simulink model "F16_Real5_OpenLoopSuccessTest_Dai3_NoHDU"  (R2016b)
settings: Solver=ode4  StartTime=0.0  StopTime=35  FixedStep=0.01  RelTol=1e-5  AbsTol=1e-4  EnableMultiTasking=on
InitFcn:
  | F16_Real5_init
libraries: simulink x2, vrlib x1
settings Model: SimulationMode=accelerator  Creator=WhisPer  LastModifiedBy=dream
settings DataIOCC: LimitDataPoints=on  SaveFormat=Array
settings OptimizationCC: LifeSpan=inf
settings DebuggingCC: UnderspecifiedInitializationDetection=Classic  MergeDetectMultiDrivingBlocksExec=none  SolverPrmCheckMsg=warning  StateNameClashWarn=warning  SFUnexpectedBacktrackingDiag=warning  SFNoUnconditionalDefaultTransitionDiag=warning  SFExecutionAtInitializationDiag=none
settings HardwareCC: ProdBitPerPointer=32  ProdBitPerSizeT=32  ProdBitPerPtrDiffT=32  ProdLargestAtomicFloat=None  ProdIntDivRoundTo=Undefined  ProdEndianess=Unspecified  ProdWordSize=32  ProdHWDeviceType=32-bit Generic
settings ModelReferenceCC: PropagateSignalLabelsOutOfModel=off
settings GRTTargetCC: TargetLangStandard=C89/C90 (ANSI)  GeneratePreprocessorConditionals=Disable all
settings ConfigComp: CovMetricSettings=dw  CovHtmlReporting=on  CovSaveCumulativeToWorkspaceVar=on  CovSaveSingleToWorkspaceVar=on  CovExternalEMLEnable=off

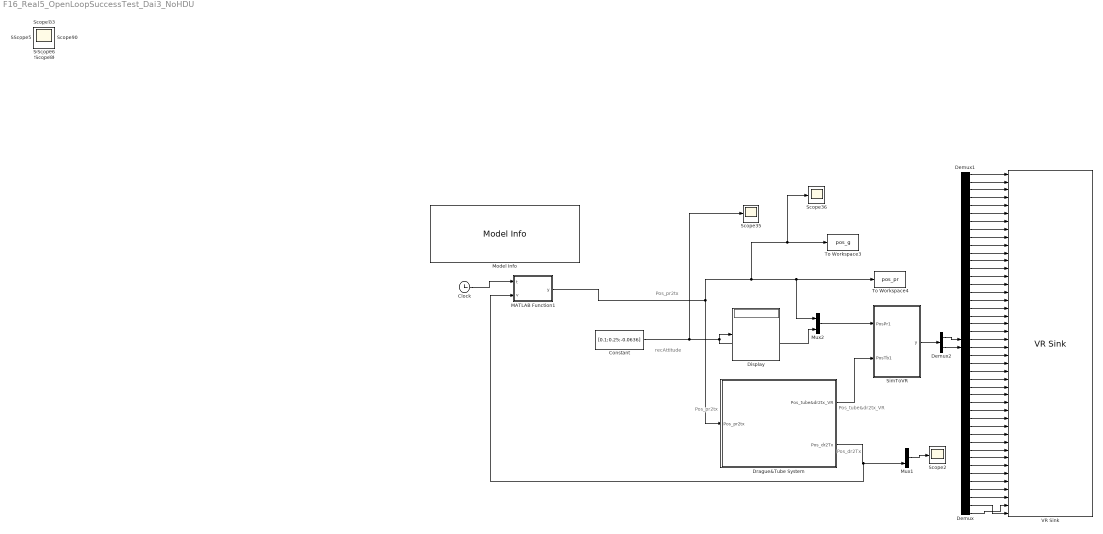
== system F16_Real5_OpenLoopSuccessTest_Dai3_NoHDU ==
  note: recAttitude
  note: Pos_dr2Tx
  note: Pos_tube&dr2tx_VR
  note: Pos_pr2tx
  note: Pos_pr2tx
  Clock : Clock
  Constant : Constant  Value=[0.1;0.25;-0.0636]
  Demux : Demux  Outputs=22
  Demux1 : Demux  Outputs=22
  Demux2 : Demux  Outputs=[88,66]
  Display : Display
  Drague&Tube System : Subsystem
      mask Display: image(imread('Icon\zhuitao.png'))
  MATLAB Function1 : MATLAB Function  TreatAsAtomicUnit=on
  Model Info : simulink/Model-Wide Utilities/Model Info  BlockCM=None  Frame=on  DisplayStringWithTags=|  HorizontalTextAlignment=Center  LeftAlignmentValue=0.5  SourceBlockDiagram=F16_Real5_OpenLoopSuccessTest_Dai3_NoHDU  TagMaxNumber=20
      | Ppr_rc=[6.06 0.54 -0.86]
      | Pns_rc=[8.00 0.00  0.00]
      | Pfl_rc=[3.75 0.00 -0.86]
      | Pdr0_tk=[-13.549 0.00 5]
  Mux1 : Mux  Inputs=2
  Mux2 : Mux  Inputs=2
  Scope{,1..36} (37 alike) : Scope
  SimToVR : MATLAB Function  TreatAsAtomicUnit=on
  To Workspace3 : ToWorkspace  VariableName=pos_g  SampleTime=-1
  To Workspace4 : ToWorkspace  VariableName=pos_pr  SampleTime=-1
  VR Sink : vrlib/VR Sink  InstantiateOnLoad=on  SampleTime=-1  ViewEnable=on  RemoteChange=off  RemoteView=off  FieldsWritten=tube1.rotation.4.1.1.double#tube1.translation.3.1.1.double#tube2.rotation.4.1.1.double#tube2.translation.3.1.1.double#tube3.rotation.4.1.1.double#tube3.translation.3.1.1.double#tube4.rotation.4.1.1.double#tube4.translation.3.1.1.double#tube5.rotation.4.1.1.double#tube5.translation.3.1.1.double#tube6.rotation.4.1.1.double#tube6.translation.3.1.1.double#tube7.rotation.4.1.1.double#tube7.translation.3.1.1.double#tube8.rotation.4.1.1.double#tube8.translation.3.1.1.double#tube9.rotation.4.1.1.double#tube9.translation.3.1.1.double#tube10.rotation.4.1.1.double#tube10.translation.3.1.1.double#tube11.rotation.4.1.1.double#tube11.translation.3.1.1.double#tube12.rotation.4.1.1.double#tube12.translation.3.1.1.double#tube13.rotation.4.1.1.double#tube13.translation.3.1.1.double#tube14.rotation.4.1.1.double#tube14.translation.3.1.1.double#tube15.rotation.4.1.1.double#tube15.translation.3.1.1.double#tube16.rotation.4.1.1.double#tube16.translation.3.1.1.double#tube17.rotation.4.1.1.double#tube17.translation.3.1.1.double#tube18.rotation.4.1.1.double#tube18.translation.3.1.1.double#tube19.rotation.4.1.1.double#tube19.translation.3.1.1.double#tube20.rotation.4.1.1.double#tube20.translation.3.1.1.double#tube21.rotation.4.1.1.double#tube21.translation.3.1.1.double#ASDD.translation.3.1.1.double#Receiver.rotation.4.1.1.double  WorldFileName=AirRefuelingTubeSim.WRL  AutoView=off  VideoDimensions=[]  AllowVariableSize=off
  wires:
  MATLAB Function1/1(y) -> Drague&Tube System/1(Pos_pr2tx), Mux2/1, To Workspace4/1, Scope36/1, To Workspace3/1
  Drague&Tube System/2(Pos_dr2Tx) -> MATLAB Function1/2(v), Mux1/2
  Mux1/1 -> Scope2/1
  Constant/1 -> Scope35/1, Display/1, Mux2/2
  Demux2/2 -> Demux/1
  SimToVR/1(y) -> Demux2/1
  Drague&Tube System/1(Pos_tube&dr2tx_VR) -> SimToVR/2(PosTb1)
  Mux2/1 -> SimToVR/1(PosPr1)
  Demux1/1 -> VR Sink/1
  Demux/1 -> VR Sink/2
  Demux1/2 -> VR Sink/3
  Demux/2 -> VR Sink/4
  Demux1/3 -> VR Sink/5
  Demux/3 -> VR Sink/6
  Demux1/4 -> VR Sink/7
  Demux/4 -> VR Sink/8
  Demux1/5 -> VR Sink/9
  Demux/5 -> VR Sink/10
  Demux1/6 -> VR Sink/11
  Demux/6 -> VR Sink/12
  Demux1/7 -> VR Sink/13
  Demux/7 -> VR Sink/14
  Demux1/8 -> VR Sink/15
  Demux/8 -> VR Sink/16
  Demux1/9 -> VR Sink/17
  Demux/9 -> VR Sink/18
  Demux1/10 -> VR Sink/19
  Demux/10 -> VR Sink/20
  Demux1/11 -> VR Sink/21
  Demux/11 -> VR Sink/22
  Demux1/12 -> VR Sink/23
  Demux/12 -> VR Sink/24
  Demux1/13 -> VR Sink/25
  Demux/13 -> VR Sink/26
  Demux1/14 -> VR Sink/27
  Demux/14 -> VR Sink/28
  Demux1/15 -> VR Sink/29
  Demux/15 -> VR Sink/30
  Demux1/16 -> VR Sink/31
  Demux/16 -> VR Sink/32
  Demux1/17 -> VR Sink/33
  Demux/17 -> VR Sink/34
  Demux1/18 -> VR Sink/35
  Demux/18 -> VR Sink/36
  Demux1/19 -> VR Sink/37
  Demux/19 -> VR Sink/38
  Demux1/20 -> VR Sink/39
  Demux/20 -> VR Sink/40
  Demux1/21 -> VR Sink/41
  Demux/21 -> VR Sink/42
  Demux/22 -> VR Sink/43
  Demux1/22 -> VR Sink/44
  Demux2/1 -> Demux1/1
  Clock/1 -> MATLAB Function1/1(t)

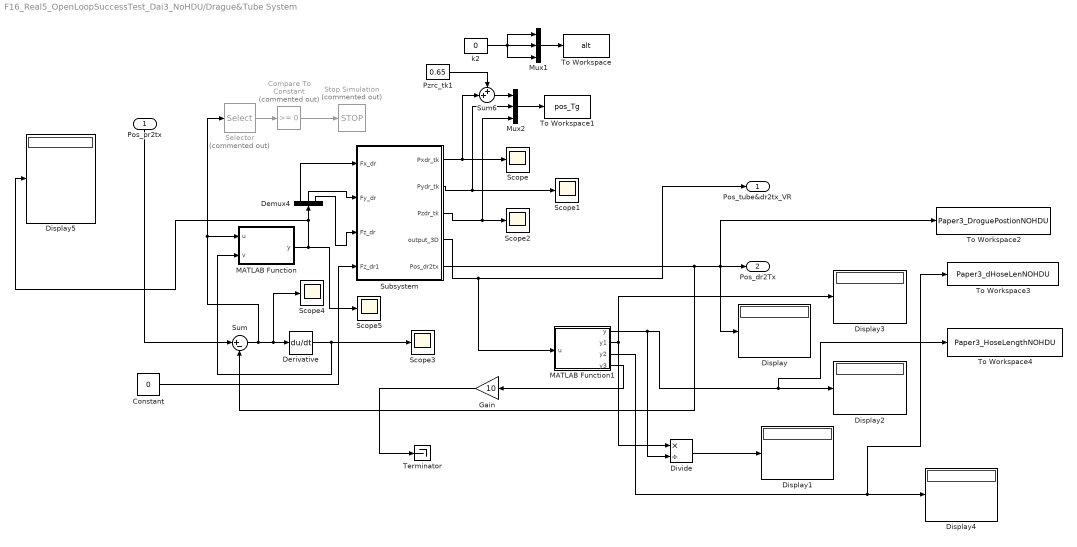
== system F16_Real5_OpenLoopSuccessTest_Dai3_NoHDU/Drague&Tube System ==
  Pos_pr2tx : Inport
  Compare To Constant : simulink/Logic and Bit Operations/Compare To Constant  Commented=on  relop=>=  const=0  OutDataTypeStr=boolean
  Constant : Constant  Value=0
  Demux4 : Demux  Outputs=3
  Derivative : Derivative
  Display{,1..5} (6 alike) : Display
  Divide : Product  Inputs=*/
  Gain : Gain  Gain=10
  MATLAB Function : MATLAB Function  TreatAsAtomicUnit=on
  MATLAB Function1 : MATLAB Function  TreatAsAtomicUnit=on
  Mux1 : Mux  Inputs=3
  Mux2 : Mux  Inputs=3
  Pzrc_tk1 : Constant  Value=0.65
  Scope{,1..5} (6 alike) : Scope
  Selector : Selector  Commented=on  InputPortWidth=3  IndexOptions=Index vector (dialog)  Indices=[1]  OutputSizes=1
  Stop Simulation : Stop  Commented=on
  Subsystem : Subsystem
  Sum : Sum  Inputs=|+-
  Sum6 : Sum  Inputs=++|
  Terminator : Terminator
  To Workspace : ToWorkspace  VariableName=alt  SampleTime=-1
  To Workspace1 : ToWorkspace  VariableName=pos_Tg  SampleTime=-1
  To Workspace2 : ToWorkspace  VariableName=Paper3_DroguePostionNOHDU  SampleTime=-1
  To Workspace3 : ToWorkspace  VariableName=Paper3_dHoseLenNOHDU  SampleTime=-1
  To Workspace4 : ToWorkspace  VariableName=Paper3_HoseLengthNOHDU  SampleTime=-1
  k2 : Constant  Value=0
  Pos_tube&dr2tx_VR : Outport
  Pos_dr2Tx : Outport  Port=2
  wires:
  Subsystem/5(Pos_dr2tx) -> Sum/2, Display/1, To Workspace2/1, Pos_dr2Tx/1
  Subsystem/3(Pzdr_tk) -> Mux2/3, Scope2/1
  Subsystem/1(Pxdr_tk) -> Scope/1, Sum6/2
  Subsystem/2(Pydr_tk) -> Mux2/2, Scope1/1
  Mux2/1 -> To Workspace1/1
  Mux1/1 -> To Workspace/1
  Pzrc_tk1/1 -> Sum6/1
  k2/1 -> Mux1/3, Mux1/1, Mux1/2
  Sum6/1 -> Mux2/1
  Subsystem/4(output_3D) -> MATLAB Function1/1(u), Pos_tube&dr2tx_VR/1
  Demux4/1 -> Subsystem/1(Fx_dr)
  Demux4/2 -> Subsystem/2(Fy_dr)
  Demux4/3 -> Subsystem/3(Fz_dr)
  Pos_pr2tx/1 -> Sum/1
  Sum/1 -> MATLAB Function/1(u), Selector/1, Scope4/1, Derivative/1
  Derivative/1 -> MATLAB Function/2(v), Scope3/1
  MATLAB Function/1(y) -> Scope5/1, Display5/1, Demux4/1
  Compare To Constant/1 -> Stop Simulation/1
  Selector/1 -> Compare To Constant/1
  MATLAB Function1/4(y3) -> Gain/1
  Gain/1 -> Terminator/1
  Constant/1 -> Subsystem/4(Fz_dr1)
  MATLAB Function1/2(y1) -> Divide/1, Display3/1
  MATLAB Function1/1(y) -> To Workspace4/1, Display2/1, Divide/2
  Divide/1 -> Display1/1
  MATLAB Function1/3(y2) -> To Workspace3/1, Display4/1

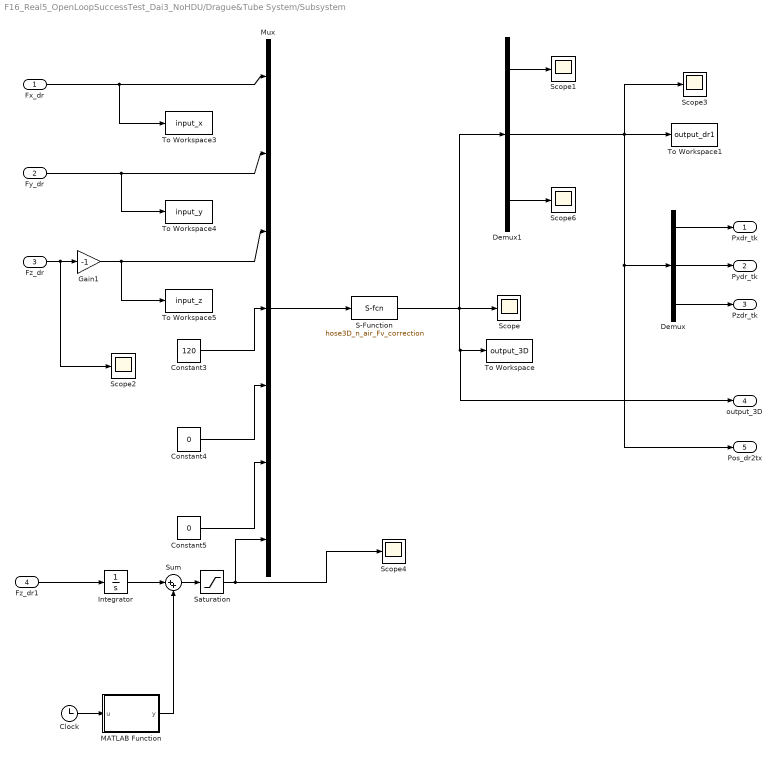
== system F16_Real5_OpenLoopSuccessTest_Dai3_NoHDU/Drague&Tube System/Subsystem ==
  Fx_dr : Inport
  Fy_dr : Inport  Port=2
  Fz_dr : Inport  Port=3
  Fz_dr1 : Inport  Port=4
  Clock : Clock
  Constant3 : Constant  Value=120
  Constant4 : Constant  Value=0
  Constant5 : Constant  Value=0
  Demux : Demux  Outputs=3
  Demux1 : Demux  Outputs=[57,3,40]
  Gain1 : Gain  Gain=-1  ParamDataTypeStr=double  OutDataTypeStr=double
  Integrator : Integrator
  MATLAB Function : MATLAB Function  TreatAsAtomicUnit=on
  Mux : Mux  Inputs=7
  S-Function : S-Function  FunctionName=hose3D_n_air_Fv_correction  SFunctionDeploymentMode=off  EnableBusSupport=off
  Saturation : Saturate  UpperLimit=13  LowerLimit=-1
  Scope{,1..4,6} (6 alike) : Scope
  Sum : Sum  Inputs=|++
  To Workspace : ToWorkspace  VariableName=output_3D  SampleTime=-1
  To Workspace1 : ToWorkspace  VariableName=output_dr1  SampleTime=-1
  To Workspace3 : ToWorkspace  VariableName=input_x  SampleTime=-1
  To Workspace4 : ToWorkspace  VariableName=input_y  SampleTime=-1
  To Workspace5 : ToWorkspace  VariableName=input_z  SampleTime=-1
  Pxdr_tk : Outport
  Pydr_tk : Outport  Port=2
  Pzdr_tk : Outport  Port=3
  output_3D : Outport  Port=4
  Pos_dr2tx : Outport  Port=5
  wires:
  Mux/1 -> S-Function/1
  Constant3/1 -> Mux/4
  Constant4/1 -> Mux/5
  Constant5/1 -> Mux/6
  Fy_dr/1 -> Mux/2, To Workspace4/1
  Fz_dr/1 -> Scope2/1, Gain1/1
  Fx_dr/1 -> To Workspace3/1, Mux/1
  Demux1/1 -> Scope1/1
  Demux1/3 -> Scope6/1
  Demux1/2 -> Pos_dr2tx/1, Demux/1, To Workspace1/1, Scope3/1
  Demux/1 -> Pxdr_tk/1
  Demux/2 -> Pydr_tk/1
  Demux/3 -> Pzdr_tk/1
  Gain1/1 -> Mux/3, To Workspace5/1
  S-Function/1 -> Demux1/1, Scope/1, output_3D/1, To Workspace/1
  Fz_dr1/1 -> Integrator/1
  Sum/1 -> Saturation/1
  Integrator/1 -> Sum/1
  Clock/1 -> MATLAB Function/1(u)
  MATLAB Function/1(y) -> Sum/2
  Saturation/1 -> Scope4/1, Mux/7

== matlab function F16_Real5_OpenLoopSuccessTest_Dai3_NoHDU/Drague&Tube System/MATLAB Function ==
  data: u input; y output; v input
function y = fcn(u,v)

persistent isXCrossBound;
if isempty(isXCrossBound)
    isXCrossBound = false;
end

persistent isRCrossBound;
if isempty(isRCrossBound)
    isRCrossBound = false;
end


persistent lastPosState;
if isempty(lastPosState)
    lastPosState = [0;0;0];
end


if ~isXCrossBound && lastPosState(1)<=0 && u(1)>0
    isXCrossBound =true;
end

if isXCrossBound&& u(1)<-0.05 && lastPosState(1) >= -0.05
    isXCrossBound=false;
end


R = sqrt(u(2)^2+u(3)^2);
RLast = sqrt(lastPosState(2)^2+lastPosState(3)^2);

RDrogue = 0.15;
% if u(1)>-0.15 && u(1)<0
%     RDrogue = 0.15*(-u(1)/0.15)+0.02;
% end


if ~isRCrossBound &&  R>(RDrogue+0.015) && u(1)>-0.1 && (u(1)<=0 || isXCrossBound) && RLast <=(RDrogue+0.01)
    isRCrossBound = true;
end

if isRCrossBound  && R<RDrogue && u(1)>-0.15 && (u(1)<=0 || isXCrossBound) && RLast>=RDrogue
    isRCrossBound = false;
end

if isRCrossBound && u(1)<=-0.15 && ~isXCrossBound
    isRCrossBound = false;
end


y=[0;0;0];


if isXCrossBound
    if u(1) <0.05
        y(1)=2000*u(1);
        if v(1)>0
            y(1) = y(1) + 1000*v(1);
        end  
    else
         y(1) = 10000*u(1);     
    end 
end

eR = R - RDrogue;
if isRCrossBound
    if eR < 0.05
        Ru = 5000*eR;
        y(2) = Ru*u(2)/R;
        y(3) = Ru*u(3)/R;
        if R>RLast
            y(2) = y(2)+ 100*v(2);
            y(3) = y(3)+ 100*v(3);
        end
    else
            Ru = 10000*eR;
            y(2) = Ru*u(2)/R;
            y(3) = Ru*u(3)/R;              
    end
end

lastPosState = u;


%y=[0;0;0];
% if u(1)<-0.1 && (u(2) > 0.05)

% if u(1)>0 && v(1)>0
% %     if v(1)>=1
% %         y(1)=1000*v(1);
% %         if(u(1)>0.05)
% %             y(1)= y(1)+10000*u(1);
% %         end
% %     else
% %         if(u(1)>0.05)
% %             y(1)=10000*u(1);
% %         else
% %             y(1)=500*u(1)+100*v(1);
% %         end 
% %     end
%     y(1)=1000*u(1);
%     if u(1)>0.01
%         y(1)=2000*u(1);
%     end
%     
%     if u(1)>0.02
%         y(1)=5000*u(1);
%     end  
%     %y(1)=y(1)+100*v(1);
%     
% end


% if u(1)>-0.1 && u(2) > 0.05 %&& u(2) <0.08
%     y(2)=5000*(u(2)-0.05);
% end
% 
% if u(1)>-0.1 && u(2) <- 0.05 %&&  u(2) >- 0.08
%     y(2)=5000*(u(2)+0.05);
% end
% 
% if u(1)>-0.1 && u(3) > 0.05 %&&  u(3) < 0.08
%     y(3)=5000*(u(3)-0.05);
% end
% 
% if u(1)>-0.1 && u(3) <- 0.05 %&& u(3) >- 0.08
%     y(3)=5000*(u(3)+0.05);
% end




% if u(1)>-0.15 && u(3) > 0.2
%     if v(3)>=1
%         y(3)=1000*v(3);
%     else
%         y(3)=5000*(u(3)-0.2)+100*v(3);
%     end
% end
% 
% if u(1)>-0.15 && u(3) <- 0.2
%     if v(3)<=-1
%         y(3)=1000*v(3);
%     else
%         y(3)=5000*(u(3)+0.2)+100*v(3);
%     end
% end

== matlab function F16_Real5_OpenLoopSuccessTest_Dai3_NoHDU/SimToVR ==
  data: y output; PosPr1 input; PosTb1 input
function y = SimToVR(PosPr1,PosTb1)
%#codegen

%%函数名：SimToVR
%%用途  ：将软管锥套坐标输出转换为VR输入
%%输入  ：PosPr - 受油机椎管坐标， PlsTb - 软管坐标数据
%%输出  ：VrPos - 软管和受油机VR位置，VrAngle - 旋转角度输出
%%作者  ：戴训华
%%时间  ：2014/3/19

PosPr = PosPr1(1:3);
AttitudeRecei = [PosPr1(4);-PosPr1(6);PosPr1(5)-0.115609];

PosTb = PosTb1(1:60);

VrAngle = zeros(22*4,1);
VrPos = zeros(22*3,1);


for j = 1:21                        %前20为软管坐标数据，后1为软管平滑过渡处理
    if j == 1
        pX = [0, 0, 0]';            %软管起点
        pY = PosTb(3*j-2:3*j);      %软杆终点
    elseif j == 21                  %多加一段杆，做过渡
        pX = PosTb(3*j-5:3*j-3);
        pY = [PosTb(3*j-5)-0.7163*cos(8/180*pi),PosTb(3*j-4),PosTb(3*j-3)+0.7163*sin(8/180*pi)]';
    else
        pX = PosTb(3*j-5:3*j-3);
        pY = PosTb(3*j-2:3*j); 
    end
    
    pZ = (pX + pY)/2;               %中点坐标
    pZ = pZ * 8/3;                  %到VR中比例的缩放

    vAxis = [0,0,-1]';               %水平轴
    vTb = pY - pX;                  %杆的方向
    
    axis1 = null([vAxis';vTb']);%获取垂直向量
    vRot = axis1(:,1)';             %得到旋转轴
    
    if vRot(2) < 0
        vRot = -vRot;
    end
    
    VrAngle(4*j-3:4*j-1) = [vRot(1),vRot(3),vRot(2)]';
    VrAngle(4*j) = acos(vAxis'*vTb / sqrt(vAxis'*vAxis * vTb'*vTb));
    
    VrPos(3*j-2:3*j) = [pZ(1),-pZ(3),pZ(2)]';
end
%y = u;
VrAngle(85:88)=[AttitudeRecei(1);AttitudeRecei(2);AttitudeRecei(3);norm(AttitudeRecei)];
pZ = PosPr+[0.25 -0.1 -0.05]';
pZ = pZ * 8/3;
VrPos(3*22-2:3*22) = [pZ(1),-pZ(3),pZ(2)]';

VrPos(3*21-2) = VrPos(3*21-2)+0.8;
VrPos(3*21-1) = VrPos(3*21-1)+0.1;

y = [VrAngle;VrPos];

== matlab function F16_Real5_OpenLoopSuccessTest_Dai3_NoHDU/Drague&Tube System/Subsystem/MATLAB Function ==
  data: u input; y output
function y = fcn(u)
if u<=8
    y=11-(u*11/8);
    
else
    y=0;
end

== matlab function F16_Real5_OpenLoopSuccessTest_Dai3_NoHDU/MATLAB Function1 ==
  data: t input; y output; v input
function y = fcn(t,v)
y=zeros(3,1);
y(1)=-13-10;
y(2)=0.02;
y(3)=5;

if t>10&&t<22
    y(1)=-13-10+(t-10)*11/12;
%     if t>=21
%         y(2)=-0.2;
%     end
end

if t>=22&&t<26
    y(1)=-13-10+(22-10)*11/12;
end
% if t>=22
%     y(2)=1;
%     y(1) = -11;
% end
if t>=26 && t<28
    y(1)=-13-10+(22-10)*11/12-(t-26)*11/2;
    %y(3)=4.9;
end

== matlab function F16_Real5_OpenLoopSuccessTest_Dai3_NoHDU/Drague&Tube System/MATLAB Function1 ==
  data: u input; y output; y1 output; y2 output; y3 output
function [y,y1,y2,y3] = fcn(u)
ll=zeros(20,1);
for i=1:20
    if i==1
       uk_1 = [0;0;0];
    else
        uk_1 = [u(3*(i-1)-2);u(3*(i-1)-2+1);u(3*(i-1)-2+2)];
    end
    uk = [u(3*(i)-2);u(3*(i)-2+1);u(3*(i)-2+2)];
    
    ll(i)=sqrt((uk(1)-uk_1(1))^2+(uk(2)-uk_1(2))^2+(uk(3)-uk_1(3))^2);
end

y = sum(ll);

y1= sqrt((u(58))^2+(u(59))^2+(u(60))^2);
y2 = y1-y;

y3  = 0;

if ((y1/14.29*14.33-y)/y) <=-0.003
    y3 = -0.2*(y1/14.29*14.33-y);
elseif ((y1/14.29*14.33-y)/y) <-0.003
    y3=sat((y-14.33)/0.2)*0.2*0.01;
end

y2=(y1/14.29*14.33-y)/y;
